simulink model "Damper"  (R2022b)
settings: Solver=VariableStepAuto  StartTime=0.0  StopTime=10.0  RelTol=1e-3
values from neighbouring files (symbols this model uses):
  b = 5    [InitDamperMass.m]
  k = 6    [InitDamperMass.m]
  m = 2    [InitDamperMass.m]
  omega = 0.5    [InitDamperMass.m]
  v0 = 0    [InitDamperMass.m]    (also in InitTwoBody.m = [3.021; 24.139; 10.964])
  x0 = 1    [InitDamperMass.m]
settings Model: Creator=filippocamaleonte  LastModifiedBy=filippocamaleonte

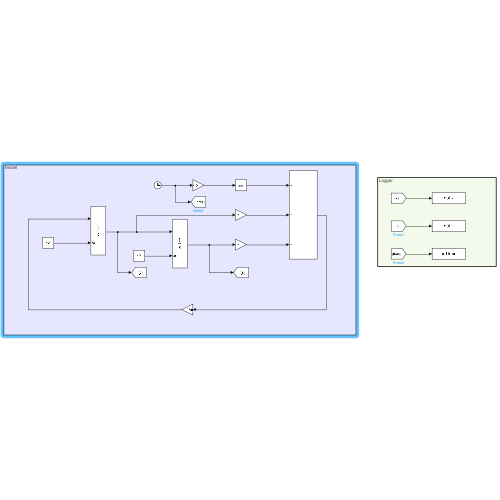
[thumbnail: Simulink's stored preview of the top-level diagram]
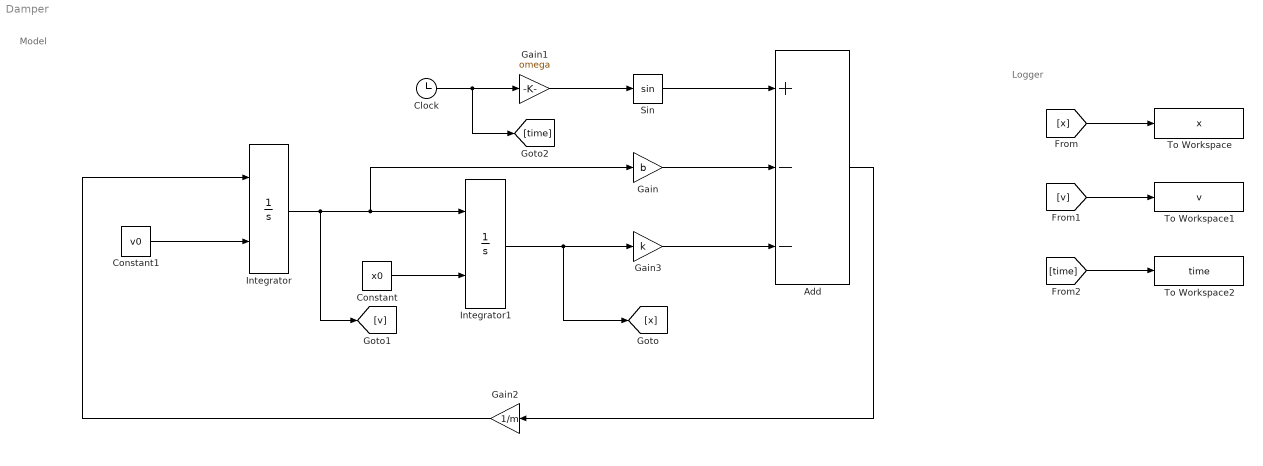
== system Damper ==
  note: Model
  note: Logger
  Add : Sum  Inputs=+--
  Clock : Clock
  Constant : Constant  Value=x0
  Constant1 : Constant  Value=v0
  Gain : Gain  Gain=b
  Gain1 : Gain  Gain=omega
  Gain2 : Gain  Gain=1/m
  Gain3 : Gain  Gain=k
  Integrator : Integrator  InitialConditionSource=external
  Integrator1 : Integrator  InitialConditionSource=external
  Sin : Trigonometry
  To Workspace : ToWorkspace  VariableName=x  SaveFormat=Timeseries  SampleTime=-1
  To Workspace1 : ToWorkspace  VariableName=v  SaveFormat=Timeseries  SampleTime=-1
  To Workspace2 : ToWorkspace  VariableName=time  SaveFormat=Timeseries  SampleTime=-1
  wires:
  Integrator/1 -> [v], Gain/1, Integrator1/1
  Constant/1 -> Integrator1/2
  Constant1/1 -> Integrator/2
  Integrator1/1 -> [x], Gain3/1
  Clock/1 -> [time], Gain1/1
  Gain1/1 -> Sin/1
  Sin/1 -> Add/1
  Gain/1 -> Add/2
  Gain3/1 -> Add/3
  Add/1 -> Gain2/1
  Gain2/1 -> Integrator/1
  [x] -> To Workspace/1
  [v] -> To Workspace1/1
  [time] -> To Workspace2/1
